simulink model "model1_sim"  (R2016a)
settings: Solver=VariableStepAuto  StartTime=0.0  StopTime=15  MaxStep=0.001  RelTol=1e-6
values from neighbouring files (symbols this model uses):
  bed_pos_initial = 0    [model1.m]
  damp_spring1 = 1000    [model1.m]
  damp_spring2 = 100    [model1.m]
  DC_delay = 0.005    [model1.m]    (also in model2.m)
  DC_max_force = 400    [model1.m]    (also in model2.m = 200)
  DC_PID_D = 0    [model1.m]    (also in model2.m = 1000)
  DC_PID_I = 0    [model1.m]    (also in model2.m)
  DC_PID_P = 0    [model1.m]    (also in model2.m)
  k_spring1 = 8000    [model1.m]
  k_spring2 = 20000    [model1.m]
  linear_act_delay = 0.1    [model1.m]    (also in model2.m)
  linear_act_max = 0.25    [model1.m]    (also in model2.m = 0.5)
  linear_act_speed = 0.1    [model1.m]    (also in model2.m)
  m_bed = 10    [model1.m]    (also in model2.m)
  m_curve = 5    [model1.m]
  m_payload = m_bed + m_patient    (= 40)    [model1.m]    (also in model2.m)
  max_offset = 0.1    [model1.m]    (also in model2.m)
  noise_rate = 0.1    [model1.m]    (also in model2.m)
  noise_start_time = 3    [model1.m]    (also in model2.m)
  patient_sit_time = 1    [model1.m]    (also in model2.m)
libraries: simulink x4
settings Model: Creator=Perttu  LastModifiedBy=Perttu
settings SolverCC: InitialStep=0.0005

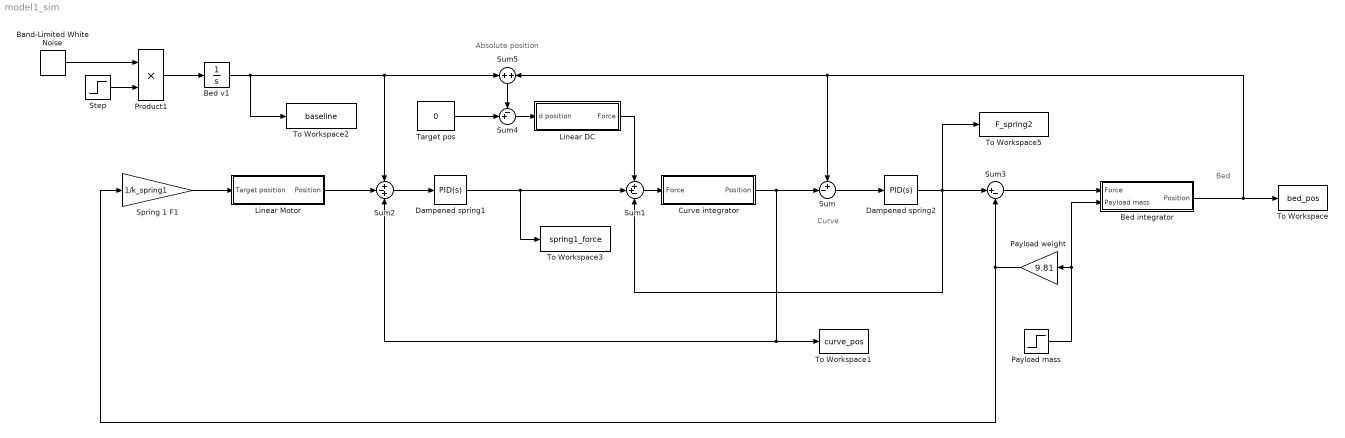
== system model1_sim ==
  note: Absolute position
  note: Curve
  note: Bed
  Band-Limited White Noise : simulink/Sources/Band-Limited White Noise  Cov=noise_power  Ts=noise_rate  seed=noise_seed
  Bed integrator : Subsystem
  Bed v1 : Integrator
  Curve integrator : Subsystem
  Dampened spring1 : simulink/Continuous/PID Controller  Controller=PID  TimeDomain=Continuous-time  SampleTime=-1  IntegratorMethod=Forward Euler  FilterMethod=Forward Euler  Form=Parallel  UseFilter=on  ControllerParametersSource=internal  P=-k_spring1  I=0  D=-damp_spring1  N=100  InitialConditionSource=internal  InitialConditionForIntegrator=0  InitialConditionForFilter=0  ExternalReset=none  LimitOutput=off  UpperSaturationLimit=inf  LowerSaturationLimit=-inf  LinearizeAsGain=on  AntiWindupMode=none  Kb=1  TrackingMode=off  Kt=1  PParamMin=[]  PParamMax=[]  IParamMin=[]  IParamMax=[]  DParamMin=[]  DParamMax=[]  NParamMin=[]  NParamMax=[]  KbParamMin=[]  KbParamMax=[]  KtParamMin=[]  KtParamMax=[]  POutMin=[]  POutMax=[]  IOutMin=[]  IOutMax=[]  DOutMin=[]  DOutMax=[]  NOutMin=[]  NOutMax=[]  KbOutMin=[]  KbOutMax=[]  KtOutMin=[]  KtOutMax=[]  IntegratorOutMin=[]  IntegratorOutMax=[]  FilterOutMin=[]  FilterOutMax=[]  SumOutMin=[]  SumOutMax=[]  SumI1OutMin=[]  SumI1OutMax=[]  SumI2OutMin=[]  SumI2OutMax=[]  SumI3OutMin=[]  SumI3OutMax=[]  SumDOutMin=[]  SumDOutMax=[]  SaturationOutMin=[]  SaturationOutMax=[]  IntegratorContinuousStateAttributes=''  IntegratorStateMustResolveToSignalObject=off  IntegratorRTWStateStorageClass=Auto  FilterContinuousStateAttributes=''  FilterStateMustResolveToSignalObject=off  FilterRTWStateStorageClass=Auto  DifferentiatorICPrevScaledInput=0  DifferentiatorOutMin=[]  DifferentiatorOutMax=[]
  Dampened spring2 : simulink/Continuous/PID Controller  Controller=PID  TimeDomain=Continuous-time  SampleTime=-1  IntegratorMethod=Forward Euler  FilterMethod=Forward Euler  Form=Parallel  UseFilter=on  ControllerParametersSource=internal  P=-k_spring2  I=0  D=-damp_spring2  N=100  InitialConditionSource=internal  InitialConditionForIntegrator=0  InitialConditionForFilter=0  ExternalReset=none  LimitOutput=off  UpperSaturationLimit=inf  LowerSaturationLimit=-inf  LinearizeAsGain=on  AntiWindupMode=none  Kb=1  TrackingMode=off  Kt=1  PParamMin=[]  PParamMax=[]  IParamMin=[]  IParamMax=[]  DParamMin=[]  DParamMax=[]  NParamMin=[]  NParamMax=[]  KbParamMin=[]  KbParamMax=[]  KtParamMin=[]  KtParamMax=[]  POutMin=[]  POutMax=[]  IOutMin=[]  IOutMax=[]  DOutMin=[]  DOutMax=[]  NOutMin=[]  NOutMax=[]  KbOutMin=[]  KbOutMax=[]  KtOutMin=[]  KtOutMax=[]  IntegratorOutMin=[]  IntegratorOutMax=[]  FilterOutMin=[]  FilterOutMax=[]  SumOutMin=[]  SumOutMax=[]  SumI1OutMin=[]  SumI1OutMax=[]  SumI2OutMin=[]  SumI2OutMax=[]  SumI3OutMin=[]  SumI3OutMax=[]  SumDOutMin=[]  SumDOutMax=[]  SaturationOutMin=[]  SaturationOutMax=[]  IntegratorContinuousStateAttributes=''  IntegratorStateMustResolveToSignalObject=off  IntegratorRTWStateStorageClass=Auto  FilterContinuousStateAttributes=''  FilterStateMustResolveToSignalObject=off  FilterRTWStateStorageClass=Auto  DifferentiatorICPrevScaledInput=0  DifferentiatorOutMin=[]  DifferentiatorOutMax=[]
  Linear DC : Subsystem
  Linear Motor : Subsystem
  Payload mass : Step  Time=patient_sit_time  Before=m_bed  After=m_payload  SampleTime=0
  Payload weight : Gain  Gain=9.81
  Product1 : Product
  Spring 1 F1 : Gain  Gain=1/k_spring1
  Step : Step  Time=noise_start_time  SampleTime=0
  Sum : Sum  Inputs=+-|
  Sum1 : Sum  Inputs=++-
  Sum2 : Sum  Inputs=+-+
  Sum3 : Sum  Inputs=|+-
  Sum4 : Sum  Inputs=-+|
  Sum5 : Sum
  Target pos : Constant  Value=0
  To Workspace : ToWorkspace  VariableName=bed_pos  SaveFormat=Timeseries  SampleTime=-1
  To Workspace1 : ToWorkspace  VariableName=curve_pos  SaveFormat=Timeseries  SampleTime=-1
  To Workspace2 : ToWorkspace  VariableName=baseline  SaveFormat=Timeseries  SampleTime=-1
  To Workspace3 : ToWorkspace  VariableName=spring1_force  SaveFormat=Timeseries  SampleTime=-1
  To Workspace5 : ToWorkspace  VariableName=F_spring2  SaveFormat=Timeseries  SampleTime=-1
  wires:
  Sum/1 -> Dampened spring2/1
  Sum1/1 -> Curve integrator/1(Force)
  Linear DC/1(Force) -> Sum1/1
  Linear Motor/1(Position) -> Sum2/2
  Curve integrator/1(Position) -> Sum/2, To Workspace1/1, Sum2/3
  Bed integrator/1(Position) -> Sum/1, Sum5/2, To Workspace/1
  Dampened spring2/1 -> Sum1/3, To Workspace5/1, Sum3/1
  Sum2/1 -> Dampened spring1/1
  Dampened spring1/1 -> Sum1/2, To Workspace3/1
  Spring 1 F1/1 -> Linear Motor/1(Target position)
  Payload weight/1 -> Spring 1 F1/1, Sum3/2
  Sum3/1 -> Bed integrator/1(Force)
  Sum4/1 -> Linear DC/1(d position)
  Target pos/1 -> Sum4/2
  Band-Limited White Noise/1 -> Product1/1
  Step/1 -> Product1/2
  Bed v1/1 -> Sum5/1, Sum2/1, To Workspace2/1
  Product1/1 -> Bed v1/1
  Payload mass/1 -> Bed integrator/2(Payload mass), Payload weight/1
  Sum5/1 -> Sum4/1

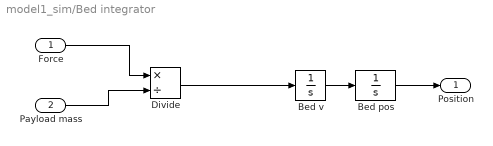
== system model1_sim/Bed integrator ==
  Force : Inport
  Payload mass : Inport  Port=2
  Bed pos : Integrator  InitialCondition=bed_pos_initial  LimitOutput=on  UpperSaturationLimit=max_offset  LowerSaturationLimit=-max_offset
  Bed v : Integrator
  Divide : Product  Inputs=*/
  Position : Outport
  wires:
  Force/1 -> Divide/1
  Bed pos/1 -> Position/1
  Bed v/1 -> Bed pos/1
  Divide/1 -> Bed v/1
  Payload mass/1 -> Divide/2

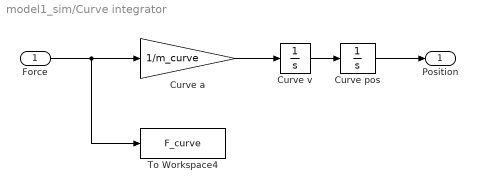
== system model1_sim/Curve integrator ==
  Force : Inport
  Curve a : Gain  Gain=1/m_curve
  Curve pos : Integrator  UpperSaturationLimit=max_offset  LowerSaturationLimit=-max_offset
  Curve v : Integrator
  To Workspace4 : ToWorkspace  VariableName=F_curve  SaveFormat=Timeseries  SampleTime=-1
  Position : Outport
  wires:
  Force/1 -> To Workspace4/1, Curve a/1
  Curve pos/1 -> Position/1
  Curve v/1 -> Curve pos/1
  Curve a/1 -> Curve v/1

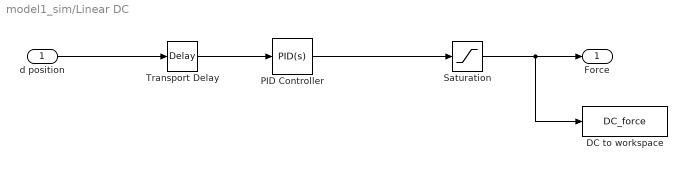
== system model1_sim/Linear DC ==
  d position : Inport
  DC to workspace : ToWorkspace  VariableName=DC_force  SaveFormat=Timeseries  SampleTime=-1
  PID Controller : simulink/Continuous/PID Controller  Controller=PID  TimeDomain=Continuous-time  SampleTime=-1  IntegratorMethod=Forward Euler  FilterMethod=Forward Euler  Form=Parallel  UseFilter=on  ControllerParametersSource=internal  P=DC_PID_P  I=DC_PID_I  D=DC_PID_D  N=100  InitialConditionSource=internal  InitialConditionForIntegrator=0  InitialConditionForFilter=0  ExternalReset=none  LimitOutput=off  UpperSaturationLimit=inf  LowerSaturationLimit=-inf  LinearizeAsGain=on  AntiWindupMode=none  Kb=1  TrackingMode=off  Kt=1  PParamMin=[]  PParamMax=[]  IParamMin=[]  IParamMax=[]  DParamMin=[]  DParamMax=[]  NParamMin=[]  NParamMax=[]  KbParamMin=[]  KbParamMax=[]  KtParamMin=[]  KtParamMax=[]  POutMin=[]  POutMax=[]  IOutMin=[]  IOutMax=[]  DOutMin=[]  DOutMax=[]  NOutMin=[]  NOutMax=[]  KbOutMin=[]  KbOutMax=[]  KtOutMin=[]  KtOutMax=[]  IntegratorOutMin=[]  IntegratorOutMax=[]  FilterOutMin=[]  FilterOutMax=[]  SumOutMin=[]  SumOutMax=[]  SumI1OutMin=[]  SumI1OutMax=[]  SumI2OutMin=[]  SumI2OutMax=[]  SumI3OutMin=[]  SumI3OutMax=[]  SumDOutMin=[]  SumDOutMax=[]  SaturationOutMin=[]  SaturationOutMax=[]  IntegratorContinuousStateAttributes=''  IntegratorStateMustResolveToSignalObject=off  IntegratorRTWStateStorageClass=Auto  FilterContinuousStateAttributes=''  FilterStateMustResolveToSignalObject=off  FilterRTWStateStorageClass=Auto  DifferentiatorICPrevScaledInput=0  DifferentiatorOutMin=[]  DifferentiatorOutMax=[]
  Saturation : Saturate  UpperLimit=DC_max_force  LowerLimit=-DC_max_force
  Transport Delay : TransportDelay  DelayTime=DC_delay  BufferSize=4096
  Force : Outport
  wires:
  Saturation/1 -> DC to workspace/1, Force/1
  PID Controller/1 -> Saturation/1
  d position/1 -> Transport Delay/1
  Transport Delay/1 -> PID Controller/1

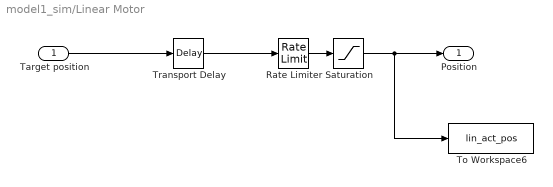
== system model1_sim/Linear Motor ==
  Target position : Inport
  Rate Limiter : RateLimiter  RisingSlewLimit=linear_act_speed  FallingSlewLimit=-linear_act_speed  SampleTimeMode=inherited  InitialCondition=m_bed * 9.81 / k_spring1
  Saturation : Saturate  UpperLimit=linear_act_max  LowerLimit=0
  To Workspace6 : ToWorkspace  VariableName=lin_act_pos  SaveFormat=Timeseries  SampleTime=-1
  Transport Delay : TransportDelay  DelayTime=linear_act_delay  InitialOutput=m_bed * 9.81 / k_spring1  BufferSize=4096
  Position : Outport
  wires:
  Target position/1 -> Transport Delay/1
  Rate Limiter/1 -> Saturation/1
  Saturation/1 -> To Workspace6/1, Position/1
  Transport Delay/1 -> Rate Limiter/1
